simulink model "robot_sim"  (R2016a)
settings: Solver=FixedStepAuto  StartTime=0.0  StopTime=10.0  FixedStep=0.001  RelTol=1e-3
libraries: simulink x4
settings Model: Creator=Shinelon  LastModifiedBy=Shinelon

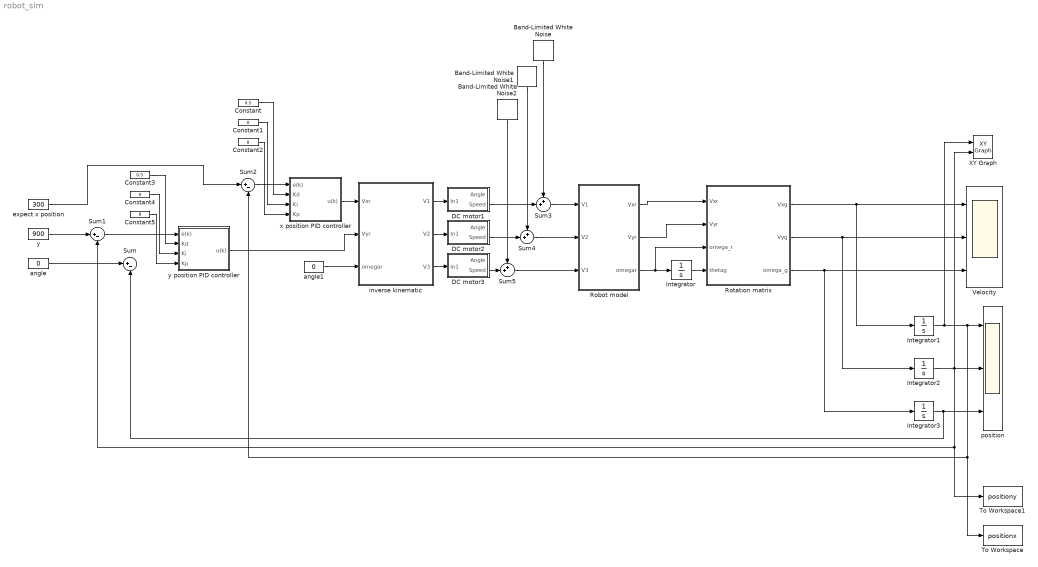
== system robot_sim ==
  Band-Limited White Noise : simulink/Sources/Band-Limited White Noise  Cov=2000  Ts=0.001  seed=[23341]
  Band-Limited White Noise1 : simulink/Sources/Band-Limited White Noise  Cov=2000  Ts=0.001  seed=[23341]
  Band-Limited White Noise2 : simulink/Sources/Band-Limited White Noise  Cov=2000  Ts=0.001  seed=[23341]
  Constant : Constant  Value=0.5
  Constant1 : Constant  Value=0
  Constant2 : Constant  Value=8
  Constant3 : Constant  Value=0.5
  Constant4 : Constant  Value=0
  Constant5 : Constant  Value=8
  DC motor1 : Subsystem
  DC motor2 : Subsystem
  DC motor3 : Subsystem
  Integrator{,1..3} (4 alike) : Integrator
  "Robot model " : MATLAB Function  TreatAsAtomicUnit=on
  "Rotation matrix " : MATLAB Function  TreatAsAtomicUnit=on
  Sum : Sum  Inputs=|+-
  Sum1 : Sum  Inputs=|+-
  Sum2 : Sum  Inputs=|+-
  Sum3 : Sum  Inputs=++|
  Sum4 : Sum  Inputs=++|
  Sum5 : Sum  Inputs=++|
  To Workspace : ToWorkspace  VariableName=positionx  SaveFormat=Timeseries  SampleTime=-1
  To Workspace1 : ToWorkspace  VariableName=positiony  SaveFormat=Timeseries  SampleTime=-1
  "Velocity " : Scope  NumInputPorts=3
  XY Graph : simulink/Sinks/XY Graph  xmin=-1000  xmax=1000  ymin=-1000  ymax=1000  st=-1
  angle : Constant  Value=0
  angle1 : Constant  Value=0
  "expect x position " : Constant  Value=300
  inverse kinematic : MATLAB Function  TreatAsAtomicUnit=on
  "position " : Scope  NumInputPorts=3
  "x position PID controller " : Subsystem
  y : Constant  Value=900
  "y position PID controller " : Subsystem
  wires:
  "Robot model "/1(Vxr) -> "Rotation matrix "/1(Vxr)
  "Robot model "/2(Vyr) -> "Rotation matrix "/2(Vyr)
  "Robot model "/3(omegar) -> "Rotation matrix "/3(omega_r), Integrator/1
  Integrator/1 -> "Rotation matrix "/4(thetag)
  "Rotation matrix "/2(Vyg) -> Integrator2/1, "Velocity "/2
  "Rotation matrix "/1(Vxg) -> Integrator1/1, "Velocity "/1
  "Rotation matrix "/3(omega_g) -> Integrator3/1, "Velocity "/3
  Integrator2/1 -> To Workspace1/1, Sum1/2, XY Graph/2, "position "/2
  Integrator1/1 -> XY Graph/1, To Workspace/1, Sum2/2, "position "/1
  Integrator3/1 -> Sum/2, "position "/3
  inverse kinematic/1(V1) -> DC motor1/1(In1)
  inverse kinematic/2(V2) -> DC motor2/1(In1)
  inverse kinematic/3(V3) -> DC motor3/1(In1)
  "expect x position "/1 -> Sum2/1
  angle/1 -> Sum/1
  y/1 -> Sum1/1
  Constant/1 -> "x position PID controller "/2("Kd ")
  Constant1/1 -> "x position PID controller "/3("Ki ")
  Constant2/1 -> "x position PID controller "/4("Kp ")
  "x position PID controller "/1(u(k)) -> inverse kinematic/1(Vxr)
  Sum2/1 -> "x position PID controller "/1(e(k))
  Constant3/1 -> "y position PID controller "/2("Kd ")
  Constant4/1 -> "y position PID controller "/3("Ki ")
  Constant5/1 -> "y position PID controller "/4("Kp ")
  Sum1/1 -> "y position PID controller "/1(e(k))
  "y position PID controller "/1(u(k)) -> inverse kinematic/2(Vyr)
  Sum3/1 -> "Robot model "/1(V1)
  DC motor1/2(Speed) -> Sum3/2
  Band-Limited White Noise/1 -> Sum3/1
  Sum4/1 -> "Robot model "/2(V2)
  DC motor2/2(Speed) -> Sum4/2
  Band-Limited White Noise1/1 -> Sum4/1
  DC motor3/2(Speed) -> Sum5/2
  Sum5/1 -> "Robot model "/3(V3)
  Band-Limited White Noise2/1 -> Sum5/1
  angle1/1 -> inverse kinematic/3(omegar)

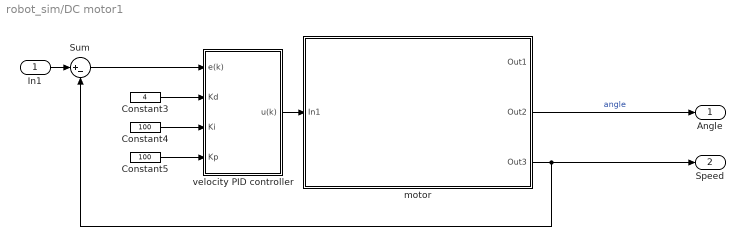
== system robot_sim/DC motor1 ==
  In1 : Inport
  Constant3 : Constant  Value=4
  Constant4 : Constant  Value=100
  Constant5 : Constant  Value=100
  Sum : Sum  Inputs=|+-
  "motor " : Subsystem  mask(DC motor subsystem){R=2, L=0.5, Km=0.1, Kf=0.2, Kemf=0.1, J=0.02}
      mask prompts: R "Resistor"; L "Inductor"; Km "Torque Constant"; Kf "Viscous Friction Constant"; Kemf "Back EMF Votage Constant"; J "Inertial Load"
      mask help:
      | This is a DC motor subsystem
      | Input : Control Signal
      | Output : Motor Rate
      mask init:
      | R=2;
      | L=0.5;
      | Km=0.1;
      | Kemf=0.1;
      | Kf=0.2;
      | J=0.02;
      mask Display:
      | color('red');port_label('input',1,'Control Signal');
      | color('red');port_label('output',1,'Torque');
      | color('red');port_label('output',2,'Angle');
      | color('red');port_label('output',3,'Speed');
      | image(imread('E:\simulink model\DC motor model\timg.jpg'))
  "velocity PID controller " : Subsystem
  "Angle " : Outport
  Speed : Outport  Port=2
  wires:
  "motor "/3(Out3) -> Speed/1, Sum/2
  "motor "/2(Out2) -> "Angle "/1  "angle"
  In1/1 -> Sum/1
  "velocity PID controller "/1(u(k)) -> "motor "/1(In1)
  Sum/1 -> "velocity PID controller "/1(e(k))
  Constant3/1 -> "velocity PID controller "/2("Kd ")
  Constant4/1 -> "velocity PID controller "/3("Ki ")
  Constant5/1 -> "velocity PID controller "/4("Kp ")

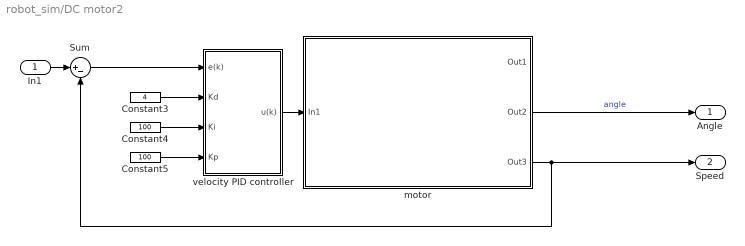
== system robot_sim/DC motor2 ==
  In1 : Inport
  Constant3 : Constant  Value=4
  Constant4 : Constant  Value=100
  Constant5 : Constant  Value=100
  Sum : Sum  Inputs=|+-
  "motor " : Subsystem  mask(DC motor subsystem){R=2, L=0.5, Km=0.1, Kf=0.2, Kemf=0.1, J=0.02}
      mask prompts: R "Resistor"; L "Inductor"; Km "Torque Constant"; Kf "Viscous Friction Constant"; Kemf "Back EMF Votage Constant"; J "Inertial Load"
      mask help:
      | This is a DC motor subsystem
      | Input : Control Signal
      | Output : Motor Rate
      mask init:
      | R=2;
      | L=0.5;
      | Km=0.1;
      | Kemf=0.1;
      | Kf=0.2;
      | J=0.02;
      mask Display:
      | color('red');port_label('input',1,'Control Signal');
      | color('red');port_label('output',1,'Torque');
      | color('red');port_label('output',2,'Angle');
      | color('red');port_label('output',3,'Speed');
      | image(imread('E:\matlab\simulink model\DC motor model\timg.jpg'))
  "velocity PID controller " : Subsystem
  "Angle " : Outport
  Speed : Outport  Port=2
  wires:
  "motor "/3(Out3) -> Speed/1, Sum/2
  "motor "/2(Out2) -> "Angle "/1  "angle"
  In1/1 -> Sum/1
  "velocity PID controller "/1(u(k)) -> "motor "/1(In1)
  Sum/1 -> "velocity PID controller "/1(e(k))
  Constant3/1 -> "velocity PID controller "/2("Kd ")
  Constant4/1 -> "velocity PID controller "/3("Ki ")
  Constant5/1 -> "velocity PID controller "/4("Kp ")

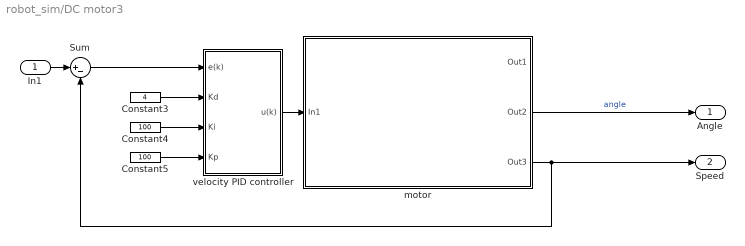
== system robot_sim/DC motor3 ==
  In1 : Inport
  Constant3 : Constant  Value=4
  Constant4 : Constant  Value=100
  Constant5 : Constant  Value=100
  Sum : Sum  Inputs=|+-
  "motor " : Subsystem  mask(DC motor subsystem){R=2, L=0.5, Km=0.1, Kf=0.2, Kemf=0.1, J=0.02}
      mask prompts: R "Resistor"; L "Inductor"; Km "Torque Constant"; Kf "Viscous Friction Constant"; Kemf "Back EMF Votage Constant"; J "Inertial Load"
      mask help:
      | This is a DC motor subsystem
      | Input : Control Signal
      | Output : Motor Rate
      mask init:
      | R=2;
      | L=0.5;
      | Km=0.1;
      | Kemf=0.1;
      | Kf=0.2;
      | J=0.02;
      mask Display:
      | color('red');port_label('input',1,'Control Signal');
      | color('red');port_label('output',1,'Torque');
      | color('red');port_label('output',2,'Angle');
      | color('red');port_label('output',3,'Speed');
      | image(imread('E:\simulink model\DC motor model\timg.jpg'))
  "velocity PID controller " : Subsystem
  "Angle " : Outport
  Speed : Outport  Port=2
  wires:
  "motor "/3(Out3) -> Speed/1, Sum/2
  "motor "/2(Out2) -> "Angle "/1  "angle"
  In1/1 -> Sum/1
  "velocity PID controller "/1(u(k)) -> "motor "/1(In1)
  Sum/1 -> "velocity PID controller "/1(e(k))
  Constant3/1 -> "velocity PID controller "/2("Kd ")
  Constant4/1 -> "velocity PID controller "/3("Ki ")
  Constant5/1 -> "velocity PID controller "/4("Kp ")

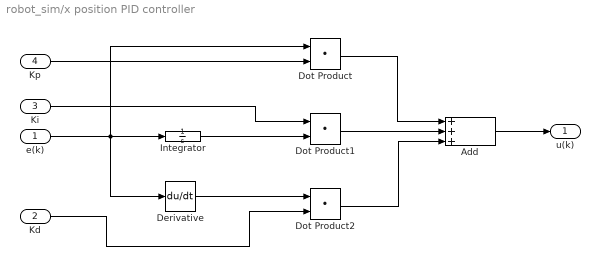
== system robot_sim/x position PID controller  ==
  e(k) : Inport
  "Kd " : Inport  Port=2
  "Ki " : Inport  Port=3
  "Kp " : Inport  Port=4
  Add : Sum  Inputs=+++
  Derivative : Derivative
  Dot Product : DotProduct  InputSameDT=on  OutDataTypeStr=Inherit: Inherit via internal rule
  Dot Product1 : DotProduct  InputSameDT=on  OutDataTypeStr=Inherit: Inherit via internal rule
  Dot Product2 : DotProduct  InputSameDT=on  OutDataTypeStr=Inherit: Inherit via internal rule
  Integrator : Integrator
  u(k) : Outport
  wires:
  "Ki "/1 -> Dot Product1/1
  "Kp "/1 -> Dot Product/2
  Add/1 -> u(k)/1
  Derivative/1 -> Dot Product2/1
  Dot Product/1 -> Add/1
  Dot Product2/1 -> Add/3
  Integrator/1 -> Dot Product1/2
  "Kd "/1 -> Dot Product2/2
  Dot Product1/1 -> Add/2
  e(k)/1 -> Dot Product/1, Integrator/1, Derivative/1

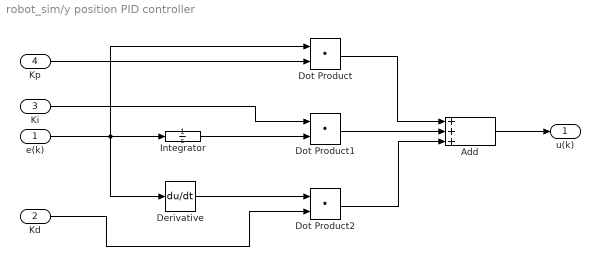
== system robot_sim/y position PID controller  ==
  e(k) : Inport
  "Kd " : Inport  Port=2
  "Ki " : Inport  Port=3
  "Kp " : Inport  Port=4
  Add : Sum  Inputs=+++
  Derivative : Derivative
  Dot Product : DotProduct  InputSameDT=on  OutDataTypeStr=Inherit: Inherit via internal rule
  Dot Product1 : DotProduct  InputSameDT=on  OutDataTypeStr=Inherit: Inherit via internal rule
  Dot Product2 : DotProduct  InputSameDT=on  OutDataTypeStr=Inherit: Inherit via internal rule
  Integrator : Integrator
  u(k) : Outport
  wires:
  "Ki "/1 -> Dot Product1/1
  "Kp "/1 -> Dot Product/2
  Add/1 -> u(k)/1
  Derivative/1 -> Dot Product2/1
  Dot Product/1 -> Add/1
  Dot Product2/1 -> Add/3
  Integrator/1 -> Dot Product1/2
  "Kd "/1 -> Dot Product2/2
  Dot Product1/1 -> Add/2
  e(k)/1 -> Dot Product/1, Integrator/1, Derivative/1

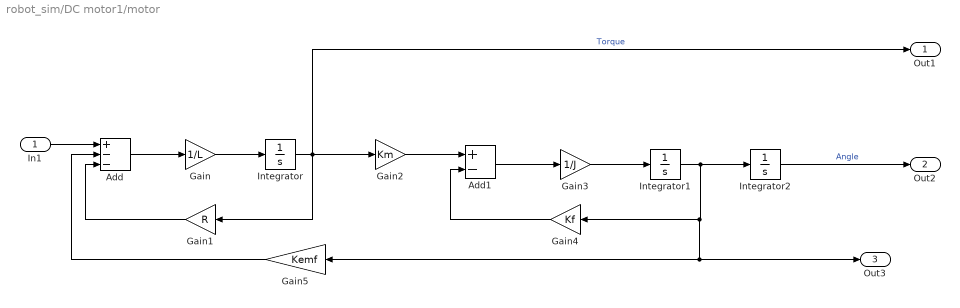
== system robot_sim/DC motor1/motor  ==
  In1 : Inport
  Add : Sum  Inputs=+--
  Add1 : Sum  Inputs=+-
  Gain : Gain  Gain=1/L
  Gain1 : Gain  Gain=R
  Gain2 : Gain  Gain=Km
  Gain3 : Gain  Gain=1/J
  Gain4 : Gain  Gain=Kf
  Gain5 : Gain  Gain=Kemf
  Integrator : Integrator
  Integrator1 : Integrator
  Integrator2 : Integrator
  Out1 : Outport
  Out2 : Outport  Port=2
  Out3 : Outport  Port=3
  wires:
  Gain5/1 -> Add/2
  Integrator/1 -> Out1/1, Gain2/1, Gain1/1  "Torque"
  Integrator2/1 -> Out2/1  "Angle"
  Add/1 -> Gain/1
  Gain/1 -> Integrator/1
  Gain1/1 -> Add/3
  Gain2/1 -> Add1/1
  Add1/1 -> Gain3/1
  Gain3/1 -> Integrator1/1
  Integrator1/1 -> Integrator2/1, Out3/1, Gain5/1, Gain4/1
  Gain4/1 -> Add1/2
  In1/1 -> Add/1

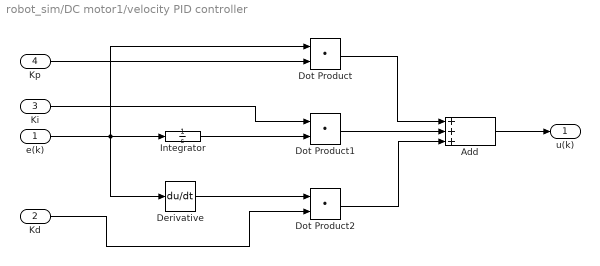
== system robot_sim/DC motor1/velocity PID controller  ==
  e(k) : Inport
  "Kd " : Inport  Port=2
  "Ki " : Inport  Port=3
  "Kp " : Inport  Port=4
  Add : Sum  Inputs=+++
  Derivative : Derivative
  Dot Product : DotProduct  InputSameDT=on  OutDataTypeStr=Inherit: Inherit via internal rule
  Dot Product1 : DotProduct  InputSameDT=on  OutDataTypeStr=Inherit: Inherit via internal rule
  Dot Product2 : DotProduct  InputSameDT=on  OutDataTypeStr=Inherit: Inherit via internal rule
  Integrator : Integrator
  u(k) : Outport
  wires:
  "Ki "/1 -> Dot Product1/1
  "Kp "/1 -> Dot Product/2
  Add/1 -> u(k)/1
  Derivative/1 -> Dot Product2/1
  Dot Product/1 -> Add/1
  Dot Product2/1 -> Add/3
  Integrator/1 -> Dot Product1/2
  "Kd "/1 -> Dot Product2/2
  Dot Product1/1 -> Add/2
  e(k)/1 -> Dot Product/1, Integrator/1, Derivative/1

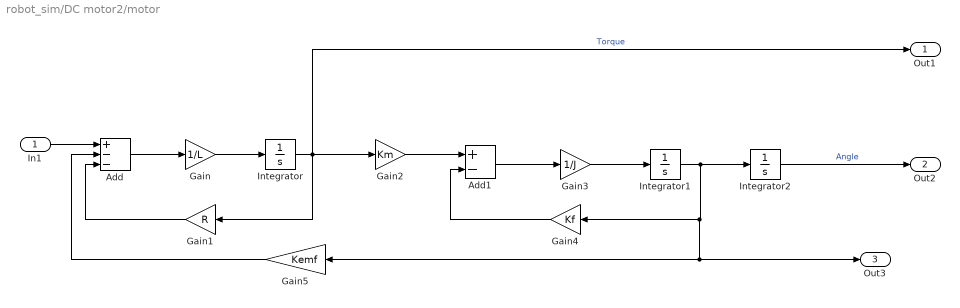
== system robot_sim/DC motor2/motor  ==
  In1 : Inport
  Add : Sum  Inputs=+--
  Add1 : Sum  Inputs=+-
  Gain : Gain  Gain=1/L
  Gain1 : Gain  Gain=R
  Gain2 : Gain  Gain=Km
  Gain3 : Gain  Gain=1/J
  Gain4 : Gain  Gain=Kf
  Gain5 : Gain  Gain=Kemf
  Integrator : Integrator
  Integrator1 : Integrator
  Integrator2 : Integrator
  Out1 : Outport
  Out2 : Outport  Port=2
  Out3 : Outport  Port=3
  wires:
  Gain5/1 -> Add/2
  Integrator/1 -> Out1/1, Gain2/1, Gain1/1  "Torque"
  Integrator2/1 -> Out2/1  "Angle"
  Add/1 -> Gain/1
  Gain/1 -> Integrator/1
  Gain1/1 -> Add/3
  Gain2/1 -> Add1/1
  Add1/1 -> Gain3/1
  Gain3/1 -> Integrator1/1
  Integrator1/1 -> Integrator2/1, Out3/1, Gain5/1, Gain4/1
  Gain4/1 -> Add1/2
  In1/1 -> Add/1

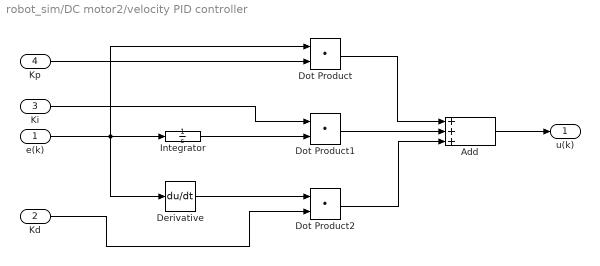
== system robot_sim/DC motor2/velocity PID controller  ==
  e(k) : Inport
  "Kd " : Inport  Port=2
  "Ki " : Inport  Port=3
  "Kp " : Inport  Port=4
  Add : Sum  Inputs=+++
  Derivative : Derivative
  Dot Product : DotProduct  InputSameDT=on  OutDataTypeStr=Inherit: Inherit via internal rule
  Dot Product1 : DotProduct  InputSameDT=on  OutDataTypeStr=Inherit: Inherit via internal rule
  Dot Product2 : DotProduct  InputSameDT=on  OutDataTypeStr=Inherit: Inherit via internal rule
  Integrator : Integrator
  u(k) : Outport
  wires:
  "Ki "/1 -> Dot Product1/1
  "Kp "/1 -> Dot Product/2
  Add/1 -> u(k)/1
  Derivative/1 -> Dot Product2/1
  Dot Product/1 -> Add/1
  Dot Product2/1 -> Add/3
  Integrator/1 -> Dot Product1/2
  "Kd "/1 -> Dot Product2/2
  Dot Product1/1 -> Add/2
  e(k)/1 -> Dot Product/1, Integrator/1, Derivative/1

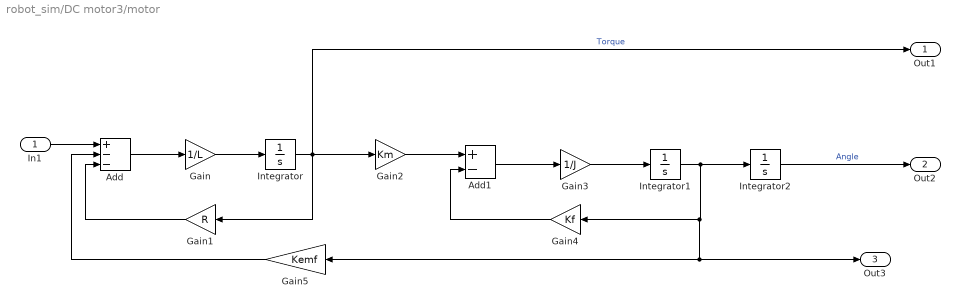
== system robot_sim/DC motor3/motor  ==
  In1 : Inport
  Add : Sum  Inputs=+--
  Add1 : Sum  Inputs=+-
  Gain : Gain  Gain=1/L
  Gain1 : Gain  Gain=R
  Gain2 : Gain  Gain=Km
  Gain3 : Gain  Gain=1/J
  Gain4 : Gain  Gain=Kf
  Gain5 : Gain  Gain=Kemf
  Integrator : Integrator
  Integrator1 : Integrator
  Integrator2 : Integrator
  Out1 : Outport
  Out2 : Outport  Port=2
  Out3 : Outport  Port=3
  wires:
  Gain5/1 -> Add/2
  Integrator/1 -> Out1/1, Gain2/1, Gain1/1  "Torque"
  Integrator2/1 -> Out2/1  "Angle"
  Add/1 -> Gain/1
  Gain/1 -> Integrator/1
  Gain1/1 -> Add/3
  Gain2/1 -> Add1/1
  Add1/1 -> Gain3/1
  Gain3/1 -> Integrator1/1
  Integrator1/1 -> Integrator2/1, Out3/1, Gain5/1, Gain4/1
  Gain4/1 -> Add1/2
  In1/1 -> Add/1

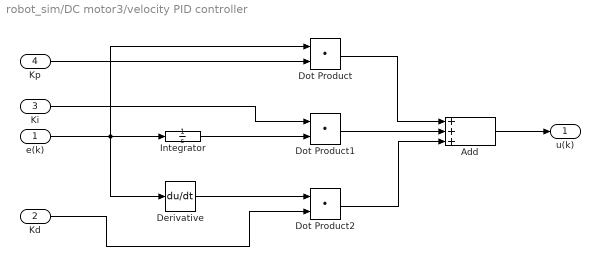
== system robot_sim/DC motor3/velocity PID controller  ==
  e(k) : Inport
  "Kd " : Inport  Port=2
  "Ki " : Inport  Port=3
  "Kp " : Inport  Port=4
  Add : Sum  Inputs=+++
  Derivative : Derivative
  Dot Product : DotProduct  InputSameDT=on  OutDataTypeStr=Inherit: Inherit via internal rule
  Dot Product1 : DotProduct  InputSameDT=on  OutDataTypeStr=Inherit: Inherit via internal rule
  Dot Product2 : DotProduct  InputSameDT=on  OutDataTypeStr=Inherit: Inherit via internal rule
  Integrator : Integrator
  u(k) : Outport
  wires:
  "Ki "/1 -> Dot Product1/1
  "Kp "/1 -> Dot Product/2
  Add/1 -> u(k)/1
  Derivative/1 -> Dot Product2/1
  Dot Product/1 -> Add/1
  Dot Product2/1 -> Add/3
  Integrator/1 -> Dot Product1/2
  "Kd "/1 -> Dot Product2/2
  Dot Product1/1 -> Add/2
  e(k)/1 -> Dot Product/1, Integrator/1, Derivative/1

== matlab function robot_sim/Rotation matrix  ==
  data: Vxr input; Vxg output; Vyr input; omega_r input; thetag input; Vyg output; omega_g output
function [Vxg,Vyg,omega_g] = Rotation(Vxr,Vyr,omega_r,thetag)
%#codegen

rotation_matrix = [cos(thetag) sin(thetag) 0
                  -sin(thetag) cos(thetag) 0
                   0           0           1];
out = rotation_matrix*[Vxr;Vyr;omega_r];
Vxg = out(1);
Vyg = out(2);
omega_g = out(3);

== matlab function robot_sim/inverse kinematic ==
  data: Vxr input; V1 output; Vyr input; omegar input; V2 output; V3 output
function [V1,V2,V3] = inverse_kinematic(Vxr,Vyr,omegar)

L = 120;
Transform_matrix = [-sqrt(3)/2 sqrt(3)/2  L;
                     1             0      L;
                    -0.5       -sqrt(3)/2 L];
input = [Vxr;Vyr;omegar];
output = Transform_matrix*input;
V1 = output(1);
V2 = output(2);
V3 = output(3);

== matlab function robot_sim/Robot model  ==
  data: V1 input; Vxr output; V2 input; V3 input; Vyr output; omegar output
function [Vxr,Vyr,omegar] = Robot(V1,V2,V3)
%#codegen
%% constant
L=120;
%% 
Transform_matrix =  [    -(2*3^(1/2))/(5*3^(1/2) + 3),       (4*3^(1/2))/(5*3^(1/2) + 3),       -(2*3^(1/2))/(5*3^(1/2) + 3);
                           6/(5*3^(1/2) + 3), (2*(3^(1/2) - 1))/(5*3^(1/2) + 3), -(2*(3^(1/2) + 2))/(5*3^(1/2) + 3);
                        (2*3^(1/2))/(3*L + 5*3^(1/2)*L), (3^(1/2) + 3)/(3*L + 5*3^(1/2)*L),    (2*3^(1/2))/(3*L + 5*3^(1/2)*L)];
Velocity = Transform_matrix*[V1;V2;V3];
Vxr = Velocity(1);
Vyr = Velocity(2);
omegar = Velocity(3);
